simulink model "FlyingSheet_simulator"  (R2019b)
settings: Solver=VariableStepAuto  StartTime=0.0  StopTime=30  RelTol=1e-3
values from neighbouring files (symbols this model uses):
  p =     [ds.mat]    (also in vxs.mat)
undefined symbols (not defined in the file or in its folder): quatnormalize
libraries: aerolibutil x24, simulink x14, sharedtransform x6, vrlib x4, sharedutil x3, simulink_extras x2, dspsrcs4 x1, aerolibanim x1, aerolibanimutils x1
(part 1 of 2)
settings Model: NumberOfSteps=10000  Creator=Robert  LastModifiedBy=Robert
settings DataIOCC: ReturnWorkspaceOutputs=off
settings DebuggingCC: ArithmeticOperatorsInVariantConditions=warning
settings SFSimCC: CustomCodeUndefinedFunction=UseInterfaceOnly

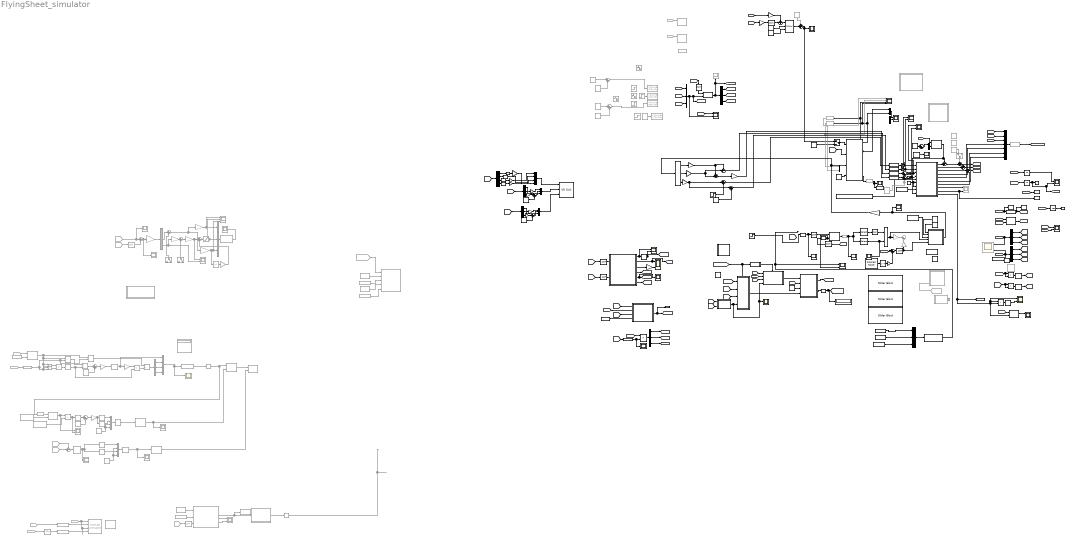
== system FlyingSheet_simulator ==
  note: Awesome Animation
  note: Green - FlyMode
      | Red = HoverMode
  note: ANimations above do not work bc gimbal lock.
  note: Thrust PID (Currently manages altitude velocity)
  note: Waypoint system,
      | Line generation,
      | reference velocity generation
  note: 0.01
  note: References are now generated in the
      |  block below this one. If you want to
      | choose your own referrence velocities
      | connect the "to" blocks with reference
      | signals here instead.
  note: Initial orientation; third argument multiplied
      | by 0 means bf and wf are aligned at start,
      | multiplied by 1 means tilted up 90 deg to
      | hiver mode at start,
  note: Man I really like playin with different reference
      | velocities, it is fun inducing crashes of the drone
  note: This is an ad-hoc way of generating a reference quaternion that can reject disturbances.
      | If body frame z-velocity is off, adjust pitch. If body frame y-velocity is off adjust yaw and roll. (This should be changed somehow)
      | body frame x-velocity is taken by another PID for joint thrust up to the right.
  note: THE HOLY GRAIL
  note: Reference velocities, set in wf
  note: For plotting trajectory in matlab
  note: Emil Fresk paper on quaternion control
  note: Rotate vector from bf to wf given q_wf
  note: Switch q between bf and wf
  note: Rotate vector from wf to bf given q_bf
  note: Matlab equivalent:
      |
      | v_wf = quatrotate(q_wf, v_bf)
      |
      |
      |
      |
      | v_bf = quatrotate(q_bf, v_wf)
      |
      |
      |
      |
      |
      |
      |
      | q_conj = quatconj(q)
  note: Adjust pitch to keep vzr_wf
  note: make sure wings horisontal
  note: See that q_uv block above? This block arangement does the same, but without calling a custom matlab block which may slow down sims.
  note: Try to figure out how to set our reference quaternion as a function of reference velocity vector, current velocity, etc.
  Abs : Abs  Commented=on
  Acos : Trigonometry  Commented=on  Operator=acos
  Acos1 : Trigonometry  Operator=acos
  AdHoc2 : MATLAB Function  Commented=on  TreatAsAtomicUnit=on
  Asin : Trigonometry  Operator=asin
  Asin1 : Trigonometry  Operator=asin
  Asin2 : Trigonometry  Operator=asin
  Band-Limited White Noise : simulink/Sources/Band-Limited White Noise  Commented=on  Cov=[0.01]  Ts=0.2  seed=[23343]
  Band-Limited White Noise1 : simulink/Sources/Band-Limited White Noise  Commented=on  Cov=[0.01]  Ts=0.1  seed=[23342]
  Band-Limited White Noise2 : simulink/Sources/Band-Limited White Noise  Commented=on  Cov=[0.01]  Ts=0.1  seed=[23341]
  Band-Limited White Noise3 : simulink/Sources/Band-Limited White Noise  Cov=[0.03]  Ts=1  seed=[23341]
  Colored Noise : dspsrcs4/Colored Noise  Color=pink  InverseFrequencyPower=1  BoundedOutput=on  NumChannels=3  OutputDataType=single  SamplesPerFrame=1  SampleTime=1/120  RandomStream=mt19937ar with seed  Seed=67  SimulateUsing=Interpreted execution
      settings: SourceProductName=DSP System Toolbox  SourceProductBaseCode=DS
  Constant : Constant  Commented=on  Value=-0.195
  Constant1 : Constant  Commented=on  Value=-5
  Constant10 : Constant  Value=6
  Constant11 : Constant  Value=15
  Constant12 : Constant  Value=0
  Constant13 : Constant  Value=18  SampleTime=p.Ts
  Constant14 : Constant  Commented=on  Value=pi/2
  Constant15 : Constant  Commented=on  Value=0
  Constant16 : Constant  Commented=on  Value=0
  Constant17 : Constant  Value=[4,8,2]'
  Constant18 : Constant  Value=0
  Constant{19..20,25..26} (4 alike) : Constant  Commented=on  Value=0.005  SampleTime=p.Ts
  Constant2 : Constant  Value=quatnormalize([cosd(60/2),0, 1*sind(60/2),0])  VectorParams1D=off
  Constant21 : Constant  Value=0
  Constant22 : Constant  Value=10
  Constant23 : Constant  Commented=on  Value=0.005*6  SampleTime=p.Ts
  Constant24 : Constant  Commented=on  Value=0.005*3  SampleTime=p.Ts
  Constant27 : Constant  Value=10
  Constant28 : Constant  Value=[4,4,10]  VectorParams1D=off
  Constant29 : Constant
  Constant3 : Constant  Value=290
  Constant30 : Constant  Value=600  SampleTime=p.Ts
  Constant31 : Constant  Value=0.6
  Constant32 : Constant  Value=0.1
  Constant4 : Constant  Commented=on  Value=-6
  Constant5 : Constant  Value=0.11  SampleTime=p.Ts
  Constant6 : Constant  Commented=on  Value=5 + 0*500
  Constant7 : Constant  Commented=on
  Constant8 : Constant
  Constant9 : Constant  Commented=on  Value=0
  Cos : Trigonometry  Commented=on  Operator=cos
  Cos1 : Trigonometry  Commented=on  Operator=cos
  Cross Product1 : vrlib/Utilities/Cross Product  Commented=on
      settings: SourceProductBaseCode=VR
  Dashboard : Subsystem
  Delay : Delay  DelayLength=1
  Demux{,2..4,6..7,10} (7 alike) : Demux  Outputs=3
  Demux1 : Demux  Commented=on  Outputs=3
  Demux5 : Demux  Commented=on  Outputs=3
  Demux8 : Demux
  Display : Display  Commented=on
  Display1 : Display
  Divide : Product  Commented=on  Inputs=*/
  Divide1 : Product  Commented=on  Inputs=*/
  Dot Product{1..3,6} (4 alike) : DotProduct  Commented=on  InputSameDT=on  OutDataTypeStr=Inherit: Inherit via internal rule
  Dot Product4 : DotProduct  InputSameDT=on  OutDataTypeStr=Inherit: Inherit via internal rule
  Dot Product5 : DotProduct  InputSameDT=on  OutDataTypeStr=Inherit: Inherit via internal rule
  Dot Product7 : DotProduct  InputSameDT=on  OutDataTypeStr=Inherit: Inherit via internal rule
  FlyVecAdjust : MATLAB Function  TreatAsAtomicUnit=on
  From : From  Commented=on  GotoTag=vr_bf
  From26 : From  Commented=on  GotoTag=q_wf
  From27 : From  Commented=on  GotoTag=vr_wf
  From28 : From  Commented=on  GotoTag=v_bf
  From33 : From  Commented=on  GotoTag=vz_wf
  From34 : From  Commented=on  GotoTag=vzr_wf
  From36 : From  Commented=on  GotoTag=r_wf
  From40 : From  Commented=on  GotoTag=q_ref
  From41 : From  Commented=on  GotoTag=r_wf
  From42 : From  Commented=on  GotoTag=q_bf
  From45 : From  Commented=on  GotoTag=hovermode
  From46 : From  Commented=on  GotoTag=hovermode
  From60 : From  Commented=on  GotoTag=q_bf
  From61 : From  Commented=on  GotoTag=q_wf
  Gain : Gain  Commented=on  Gain=30
  Gain1 : Gain  Commented=on  Gain=7.5
  Gain10 : Gain  Gain=750
  Gain11 : Gain  Commented=on  Gain=0.1
  Gain12 : Gain  Commented=on  Gain=0.02
  Gain13 : Gain
  Gain{14,16,19..20,23..27} (9 alike) : Gain  Gain=-1
  Gain15 : Gain  Commented=on  Gain=0.5
  Gain17 : Gain  Gain=10
  Gain2 : Gain  Commented=on  Gain=5
  Gain22 : Gain  Gain=-2
  Gain28 : Gain  Gain=0.1
  Gain3 : Gain
  Gain4 : Gain  Gain=0.01
  Gain5 : Gain  Commented=on  Gain=-1
  Gain6 : Gain  Commented=on  Gain=0
  Gain7 : Gain  Commented=on  Gain=0.5
  Gain8 : Gain  Commented=on  Gain=0.5
  Gain9 : Gain  Commented=on  Gain=2
  Integrator : Integrator
  Integrator1 : Integrator
  Integrator2 : Integrator
  Inveter : Subsystem
  MATLAB Animation : aerolibanim/MATLAB Animation  Tag=Matlab Animation 6 DOF  Commented=on  Vehicles=2  Geometries={'astredwedge.mat',a}  BoundingBoxCoordinates=[-50,50,-50,50,-50,50]  CameraOffset=[-150,0,0]  CameraViewAngle=3  SampleTime=0.05  FigurePosition=[962,42,958,461]
      settings: SourceProductName=Aerospace Blockset  SourceProductBaseCode=AE
  MATLAB Function : MATLAB Function  Commented=on  TreatAsAtomicUnit=on
  MATLAB Function1 : MATLAB Function  Commented=on  TreatAsAtomicUnit=on
  MATLAB Function11 : MATLAB Function  TreatAsAtomicUnit=on
  MATLAB Function12 : MATLAB Function  Commented=on  TreatAsAtomicUnit=on
  MATLAB Function2 : MATLAB Function  Commented=through  TreatAsAtomicUnit=on
  MATLAB Function3 : MATLAB Function  TreatAsAtomicUnit=on
  MATLAB Function5 : MATLAB Function  Commented=on  TreatAsAtomicUnit=on
  MATLAB Function7 : MATLAB Function  Commented=on  TreatAsAtomicUnit=on
  MATLAB Function9 : MATLAB Function  TreatAsAtomicUnit=on
  Manual Switch : ManualSwitch  Commented=on
  Manual Switch1 : ManualSwitch  Commented=on  CurrentSetting=0
  Manual Switch2 : ManualSwitch  Commented=on  CurrentSetting=0
  Manual Switch3 : ManualSwitch
  Multiply : Product
  Multiply1 : Product
  Multiply2 : Product  Commented=on
  Multiply3 : Product  Commented=on
  Mux : Mux  Inputs=7
  Mux1 : Mux  Commented=on  Inputs=3
  Mux{2,6,10,12,14} (5 alike) : Mux  Inputs=3
  Mux13 : Mux
  Mux3 : Mux  Inputs=2
  Mux4 : Mux  Inputs=2
  Mux5 : Mux  Commented=on
  Mux7 : Mux  Inputs=2
  Mux8 : Mux  Commented=on
  Mux9 : Mux  Commented=on
  Normalize Vector : vrlib/Utilities/Normalize Vector  Commented=on  maxzero=0
      settings: SourceProductName=Simulink 3D Animation  SourceProductBaseCode=VR
  Normalize Vector1 : vrlib/Utilities/Normalize Vector  maxzero=0
      settings: SourceProductName=Simulink 3D Animation  SourceProductBaseCode=VR
  PID Controller : simulink/Continuous/PID Controller  Controller=PID  Form=Parallel  TimeDomain=Discrete-time  SampleTime=-1  IntegratorMethod=Forward Euler  FilterMethod=Forward Euler  ControllerParametersSource=internal  P=3  I=3  D=0  UseFilter=off  N=100  TunerSelectOption=Frequency Response Based  InitialConditionSource=external  InitialConditionForIntegrator=0  InitialConditionForFilter=0  DifferentiatorICPrevScaledInput=0  ExternalReset=none  TrackingMode=off  Kt=1  LimitOutput=on  UpperSaturationLimit=30  LowerSaturationLimit=0  LinearizeAsGain=on  AntiWindupMode=clamping  Kb=1  POutMin=[]  POutMax=[]  IOutMin=[]  IOutMax=[]  DOutMin=[]  DOutMax=[]  NOutMin=[]  NOutMax=[]  SumOutMin=[]  SumOutMax=[]  SaturationOutMin=[]  SaturationOutMax=[]  PParamMin=[]  PParamMax=[]  IParamMin=[]  IParamMax=[]  DParamMin=[]  DParamMax=[]  NParamMin=[]  NParamMax=[]  KbParamMin=[]  KbParamMax=[]  KtParamMin=[]  KtParamMax=[]  KbOutMin=[]  KbOutMax=[]  KtOutMin=[]  KtOutMax=[]  IntegratorOutMin=[]  IntegratorOutMax=[]  FilterOutMin=[]  FilterOutMax=[]  SumI1OutMin=[]  SumI1OutMax=[]  SumI2OutMin=[]  SumI2OutMax=[]  SumI3OutMin=[]  SumI3OutMax=[]  SumI4OutMin=[]  SumI4OutMax=[]  SumDOutMin=[]  SumDOutMax=[]  DifferentiatorOutMin=[]  DifferentiatorOutMax=[]  FilterDiffOutCoefMin=[]  FilterDiffOutCoefMax=[]  ReciprocalOutMin=[]  ReciprocalOutMax=[]  SumDenOutMin=[]  SumDenOutMax=[]  SumNumOutMin=[]  SumNumOutMax=[]  DivideOutMin=[]  DivideOutMax=[]  IntegratorContinuousStateAttributes=''  IntegratorStateMustResolveToSignalObject=off  IntegratorRTWStateStorageClass=Auto  FilterContinuousStateAttributes=''  FilterStateMustResolveToSignalObject=off  FilterRTWStateStorageClass=Auto  ParallelPVariant=InternalParameters  IdealPVariant=Disabled  IVariant=InternalParameters  DVariant=InternalParameters  IntegratorVariant=Discrete  SatVariant=Enabled  AWVariant=DiscClampingParallel  PCopyVariant=Disabled  TRVariant=Disabled  FdbkBlocksVariant=Forward  IdealPFdbkVariant=Disabled  SatFdbkVariant=Disabled  DerivativeFilterVariant=Differentiator  NVariant=Passthrough  NCopyVariant=Disabled_SignalSpec  FilterICVariant=ExternalICs  IntegratorICVariant=ExternalICs  ExternalResetVariant=Disabled  TRSumVariant=Passthrough  SumFdbkVariant=Disabled  SumVariant=Sum_PID
  PID Controller5 : simulink/Continuous/PID Controller  Commented=on  Controller=PID  Form=Parallel  TimeDomain=Continuous-time  SampleTime=-1  IntegratorMethod=Forward Euler  FilterMethod=Forward Euler  ControllerParametersSource=internal  P=0.04*2  I=0  D=0  UseFilter=on  N=100  TunerSelectOption=Transfer Function Based (PID Tuner App)  InitialConditionSource=internal  InitialConditionForIntegrator=0  InitialConditionForFilter=0  DifferentiatorICPrevScaledInput=0  ExternalReset=none  TrackingMode=off  Kt=1  LimitOutput=off  UpperSaturationLimit=inf  LowerSaturationLimit=-inf  LinearizeAsGain=on  AntiWindupMode=none  Kb=1  POutMin=[]  POutMax=[]  IOutMin=[]  IOutMax=[]  DOutMin=[]  DOutMax=[]  NOutMin=[]  NOutMax=[]  SumOutMin=[]  SumOutMax=[]  SaturationOutMin=[]  SaturationOutMax=[]  PParamMin=[]  PParamMax=[]  IParamMin=[]  IParamMax=[]  DParamMin=[]  DParamMax=[]  NParamMin=[]  NParamMax=[]  KbParamMin=[]  KbParamMax=[]  KtParamMin=[]  KtParamMax=[]  KbOutMin=[]  KbOutMax=[]  KtOutMin=[]  KtOutMax=[]  IntegratorOutMin=[]  IntegratorOutMax=[]  FilterOutMin=[]  FilterOutMax=[]  SumI1OutMin=[]  SumI1OutMax=[]  SumI2OutMin=[]  SumI2OutMax=[]  SumI3OutMin=[]  SumI3OutMax=[]  SumI4OutMin=[]  SumI4OutMax=[]  SumDOutMin=[]  SumDOutMax=[]  DifferentiatorOutMin=[]  DifferentiatorOutMax=[]  FilterDiffOutCoefMin=[]  FilterDiffOutCoefMax=[]  ReciprocalOutMin=[]  ReciprocalOutMax=[]  SumDenOutMin=[]  SumDenOutMax=[]  SumNumOutMin=[]  SumNumOutMax=[]  DivideOutMin=[]  DivideOutMax=[]  IntegratorContinuousStateAttributes=''  IntegratorStateMustResolveToSignalObject=off  IntegratorRTWStateStorageClass=Auto  FilterContinuousStateAttributes=''  FilterStateMustResolveToSignalObject=off  FilterRTWStateStorageClass=Auto  ParallelPVariant=InternalParameters  IdealPVariant=Disabled  IVariant=InternalParameters  DVariant=InternalParameters  IntegratorVariant=Continuous  SatVariant=Disabled  AWVariant=Passthrough  PCopyVariant=Disabled  TRVariant=Disabled  FdbkBlocksVariant=Forward  IdealPFdbkVariant=Disabled  SatFdbkVariant=Disabled  DerivativeFilterVariant=ContFilter  NVariant=InternalParameters  NCopyVariant=Disabled  FilterICVariant=InternalICsFilter  IntegratorICVariant=InternalICs  ExternalResetVariant=Disabled  TRSumVariant=Passthrough  SumFdbkVariant=Disabled  SumVariant=Sum_PID
  Pulse Generator : DiscretePulseGenerator  Commented=on  PulseType=Time based  Amplitude=12  Period=50  PulseWidth=50
  Pulse Generator1 : DiscretePulseGenerator  Commented=on  PulseType=Time based  Amplitude=8  Period=60  PulseWidth=50  PhaseDelay=30
  Quaternion Conjugate{1..2,4..6,9} (6 alike) : aerolibutil/Quaternion Conjugate  Commented=on
      settings: SourceProductName=Aerospace Blockset  SourceProductBaseCode=AE
  Quaternion Conjugate10 : aerolibutil/Quaternion Conjugate  Commented=through
      settings: SourceProductName=Aerospace Blockset  SourceProductBaseCode=AE
  Quaternion Conjugate3 : aerolibutil/Quaternion Conjugate
      settings: SourceProductName=Aerospace Blockset  SourceProductBaseCode=AE
  Quaternion Conjugate7 : aerolibutil/Quaternion Conjugate
      settings: SourceProductName=Aerospace Blockset  SourceProductBaseCode=AE
  Quaternion Conjugate8 : aerolibutil/Quaternion Conjugate
      settings: SourceProductName=Aerospace Blockset  SourceProductBaseCode=AE
  Quaternion Multiplication : aerolibutil/Quaternion Multiplication
  Quaternion Multiplication1 : aerolibutil/Quaternion Multiplication  Commented=on
  Quaternion Multiplication2 : aerolibutil/Quaternion Multiplication  Commented=on
  Quaternion Normalize : sharedutil/Quaternion Normalize  Commented=on  aMode=aMode
      settings: SourceProductName=Aerospace Blockset  SourceProductBaseCode=AE
  Quaternion Normalize1 : sharedutil/Quaternion Normalize  Commented=on  aMode=aMode
      settings: SourceProductName=Aerospace Blockset  SourceProductBaseCode=AE
  Quaternion Normalize2 : sharedutil/Quaternion Normalize  Commented=on  aMode=aMode
      settings: SourceProductName=Aerospace Blockset  SourceProductBaseCode=AE
  Quaternion Rotation{1,4,6,8} (4 alike) : aerolibutil/Quaternion Rotation
  Quaternion Rotation{2..3,5,7} (4 alike) : aerolibutil/Quaternion Rotation  Commented=on
  Quaternions to Rotation Angles1 : sharedtransform/Quaternions to Rotation Angles  Commented=on  rotationOrder=XYZ  aMode=aMode
      settings: SourceProductBaseCode=AE
  Quaternions to Rotation Angles2 : sharedtransform/Quaternions to Rotation Angles  Commented=on  rotationOrder=XYZ  aMode=aMode
      settings: SourceProductBaseCode=AE
  Rate Limiter : RateLimiter  SampleTimeMode=inherited  InitialCondition=0.01
  Rotation Angles to Quaternions : sharedtransform/Rotation Angles to Quaternions  Commented=on  rotationOrder=ZYX  aMode=aMode
      settings: SourceProductName=Aerospace Blockset  SourceProductBaseCode=AE
  Rotation Angles to Quaternions1 : sharedtransform/Rotation Angles to Quaternions  rotationOrder=ZYX  aMode=aMode
      settings: SourceProductName=Aerospace Blockset  SourceProductBaseCode=AE
  Saturation : Saturate  UpperLimit=1000  LowerLimit=0
  Saturation1 : Saturate  UpperLimit=1000  LowerLimit=0
  Saturation2 : Saturate
  Saturation3 : Saturate
  Saturation4 : Saturate  Commented=through
  Saturation6 : Saturate  Commented=on  UpperLimit=1  LowerLimit=-1
  Scope{,2,6,10,19,23} (6 alike) : Scope  NumInputPorts=2
  Scope{1,11..12,15,18} (5 alike) : Scope  Commented=on  NumInputPorts=2
  Scope{4..5,13,20,24..26,28,34..35} (10 alike) : Scope
  Scope{3,8..9,14,17,21} (6 alike) : Scope  Commented=on
  Scope16 : Scope  Commented=on  NumInputPorts=3
  Scope27 : Scope  NumInputPorts=4
  Selector : Selector  IndexMode=Zero-based  InputPortWidth=4  IndexOptions=Index vector (dialog)  Indices=[0 ]  OutputSizes=1
  Selector1 : Selector  IndexMode=Zero-based  InputPortWidth=4  IndexOptions=Index vector (dialog)  Indices=[1:3]  OutputSizes=1
  Sign : Signum
  Signal Specification{,1..3} (4 alike) : SignalSpecification  Dimensions=1
  Signal Specification4 : SignalSpecification  Commented=through  Dimensions=14
  Signal Specification5 : SignalSpecification  Commented=through  Dimensions=[1 3]
  Simulation Pace : aerolibanimutils/Simulation Pace  Commented=on  SimulationPace=1  SleepMode=Auto  OutputPaceError=off  SampleTime=1/30
  Sin : Trigonometry  Commented=on
  Sin1 : Trigonometry  Commented=on
  Sine Wave : Sin  Commented=on  Amplitude=-2  Frequency=1/15  Phase=pi/2  SampleTime=0
  Sine Wave1 : Sin  Commented=on  Amplitude=-8  Frequency=1/20  SampleTime=0
  Sine Wave2 : Sin  Commented=on  Amplitude=10  Frequency=1/45  SampleTime=0
  Slider : SliderBlock  ScaleMin=-3.1400000000000001  ScaleMax=3.1400000000000001
  Slider1 : SliderBlock  ScaleMin=-3.1400000000000001  ScaleMax=3.1400000000000001
  Slider2 : SliderBlock  ScaleMin=-3  ScaleMax=3
  Sqrt : Sqrt  Commented=on  SaturateOnIntegerOverflow=on
  Sqrt1 : Sqrt  Commented=on  SaturateOnIntegerOverflow=on
  Sqrt2 : Sqrt  SaturateOnIntegerOverflow=on
  Sqrt3 : Sqrt  SaturateOnIntegerOverflow=on
  Sqrt4 : Sqrt  SaturateOnIntegerOverflow=on
  State-Space1 : StateSpace  Commented=on  A=-1/5  B=1/5  D=0  InitialCondition=0
  State-Space2 : StateSpace  Commented=on  A=-1/15  B=1/15  D=0  InitialCondition=0
  State-Space3 : StateSpace  Commented=on  A=-1/15  B=1/15  D=0  InitialCondition=0
  State-Space4 : StateSpace  Commented=on  A=-1/15  B=1/15  D=0  InitialCondition=0
  Step : Step  Time=20  Before=[cos(pi/4),0,sin(pi/4),0]  After=[1,0,0,0]  SampleTime=0
  Step1 : Step  Commented=on  Time=20  After=-10  SampleTime=0
  Step2 : Step  Commented=on  Time=100  After=5  SampleTime=0
  Step3 : Step  Commented=on  Time=30  Before=-1  After=0  SampleTime=0
  Step4 : Step  Commented=on  Time=60  After=18  SampleTime=0
  Step5 : Step  Time=5  Before=600  After=580  SampleTime=0
  Sum : Sum  Commented=on  Inputs=|--
  Sum{1..2,6,17..18,23,25} (7 alike) : Sum  Inputs=|++
  Sum10 : Sum  Commented=on  Inputs=|+-
  Sum{5,11..13,20} (5 alike) : Sum  Inputs=++|
  Sum{3,7..9,14..15} (6 alike) : Sum  Commented=on  Inputs=|++
  Sum16 : Sum  Inputs=-+|
  Sum19 : Sum  Inputs=-+|
  Sum21 : Sum  Commented=on  Inputs=|+-
  Sum22 : Sum  Commented=on  Inputs=-+|
  Sum24 : Sum  Inputs=|-+
  Sum4 : Sum  Inputs=+-|
  TailSitter : Subsystem
  To Workspace : ToWorkspace  VariableName=r  SaveFormat=Timeseries  SampleTime=p.Ts_log
  To Workspace1 : ToWorkspace  VariableName=q_bf  SaveFormat=Timeseries  SampleTime=p.Ts_log
  To Workspace10 : ToWorkspace  VariableName=eq_gains  SaveFormat=Timeseries  SampleTime=-1
  To Workspace2 : ToWorkspace  VariableName=v_bf  SaveFormat=Timeseries  SampleTime=p.Ts_log
  To Workspace3 : ToWorkspace  VariableName=a_bf  SaveFormat=Timeseries  SampleTime=p.Ts_log
  To Workspace4 : ToWorkspace  VariableName=q_wf  SaveFormat=Timeseries  SampleTime=p.Ts_log
  To Workspace5 : ToWorkspace  VariableName=rr  SaveFormat=Timeseries  SampleTime=p.Ts_log
  To Workspace6 : ToWorkspace  VariableName=gravity_bf  SaveFormat=Timeseries  SampleTime=p.Ts_log
  To Workspace7 : ToWorkspace  VariableName=v_wf  SaveFormat=Timeseries  SampleTime=p.Ts_log
  To Workspace8 : ToWorkspace  VariableName=refvec  SaveFormat=Timeseries  SampleTime=p.Ts_log
  To Workspace9 : ToWorkspace  Commented=on  VariableName=refvec1  SaveFormat=Timeseries  SampleTime=p.Ts_log
  TorqueTranslator : MATLAB Function  TreatAsAtomicUnit=on
  Torque_FL : MATLAB Function  Commented=on  TreatAsAtomicUnit=on
  Transfer Fcn First Order : simulink/Discrete/Transfer Fcn First Order  Commented=on  PoleZ=0.95  ICPrevOutput=0.0  DoSatur=off
      settings: SourceProductName=Simulink
  Transfer Fcn First Order1 : simulink/Discrete/Transfer Fcn First Order  Commented=on  PoleZ=0.95  ICPrevOutput=0.0  DoSatur=off
      settings: SourceProductName=Simulink
  Transpose : Math  Operator=transpose  SignedPower=off  SaturateOnIntegerOverflow=on
  VR Sink : vrlib/VR Sink  InstantiateOnLoad=on  SampleTime=0.05  ViewEnable=on  RemoteChange=off  RemoteView=off  FieldsWritten=Plane.rotation.4.1.1.double#Plane.translation.3.1.1.double#Block.translation.3.1.1.double  WorldFileName=vrtkoff_hud.wrl  WorldDescription=VR Plane Take-Off with HUD Text  AutoView=on  VideoDimensions=[600 860]  AllowVariableSize=off  FigureProperties="{'Position', 'Name', 'Viewpoint', 'CameraBound', 'CameraDirection', 'CameraPosition', 'CameraUpVector', 'ZoomFactor', 'Antialiasing', 'Headlight', 'Lighting', 'NavPanel', 'Sound', 'StatusBar', 'Stereo3D', 'Stereo3DCameraOffset', 'Stereo3DHIT', 'ToolBar', 'Textures', 'Transparency', 'Triad', 'Wireframe', 'NavZones', 'NavMode', 'NavSpeed', 'CaptureFileFormat', 'CaptureFileName', 'Record2DCompressMethod', 'Record2DCompressQuality', 'Record2D', 'Record2DFileName', 'Record2DFPS'; [9.6200000000000000e+02   8.4000000000000000e+01   9.5800000000000000e+02   3.8400000000000000e+02], 'VR Plane Take-Off with HUD Text', 'Observe Plane', 'on', [-4.2787674820401950e-01  -1.1740140648252211e-01   8.9617989159671219e-01], [1.7670687419247848e+01   7.2326607669184346e+00  -4.4972995858895132e+01], [4.6581268753260749e-03   9.9122851822676961e-01   1.3207697190645110e-01], [1.0000000000000000e+00], 'off', 'on', 'on', 'halfbar', 'on', 'on', 'off', [1.0000000149011612e-01], [0.0000000000000000e+00], 'on', 'on', 'on', 'none', 'off', 'off', 'fly', 'normal', 'tif', '%f_anim_%n.tif', 'auto', [7.5000000000000000e+01], 'off', '%f_anim_%n.avi', 'auto'}"
      settings: SourceProductBaseCode=VR
  Zero-Order Hold{,1,4..5,7..9} (7 alike) : ZeroOrderHold  SampleTime=p.Ts
  Zero-Order Hold10 : ZeroOrderHold  Commented=on  SampleTime=p.Ts
  Zero-Order Hold2 : ZeroOrderHold  Commented=on  SampleTime=p.Ts
  Zero-Order Hold6 : ZeroOrderHold  Commented=on  SampleTime=p.Ts
  bodyfrme : Scope  NumInputPorts=2
  gravity : Scope  NumInputPorts=2
  gravity_wf_convertedfrombf : Scope  NumInputPorts=2
  linegenerator : MATLAB Function  TreatAsAtomicUnit=on
  linegenerator1 : MATLAB Function  Commented=on  TreatAsAtomicUnit=on
  pitch : Constant  Value=0
  q_fly_generator : Subsystem
  q_hover_generator : Subsystem
  roll : Constant  Value=0
  u_deltas : Scope  NumInputPorts=2
  u_omegas : Scope  NumInputPorts=2
  v_isnit : Constant  Value=[0, 0,0]
  "v_ref_bf_attctrl " : Scope  Commented=on
  vr-v : Scope  Commented=on
  x_bf : Constant  Commented=on  Value=[1,0,0]
  y_bf : Constant  Commented=on  Value=[0,1,0]
  yaw : Constant  Value=0
  z_wf : Constant  Commented=on  Value=[0,0,1]
  wires:
  Selector1/1 -> Multiply/2, Scope4/1  "axiserr"
  Selector/1 -> Sign/1  "q0"
  Sign/1 -> Multiply/1  "rotdir"
  Gain1/1 -> Sum/2
  Sum5/1 -> Manual Switch3/1, Scope13/1  "u_EnginePower"
  Constant3/1 -> TailSitter/7(omegaR_init), TailSitter/6(omegaL_init)
  Sum11/1 -> [v_bf]  "v"
  TailSitter/8(wdot) -> Scope1/1  "wdot"
  TailSitter/9(vdot) -> To Workspace3/1, Scope1/2  "vdot"
  Integrator/1 -> [r_wf], Scope2/2, To Workspace/1  "r_wf"
  [v_wf] -> Integrator/1
  v_isnit/1 -> TailSitter/8(v_init)
  Sum4/1 -> PID Controller/1
  PID Controller/1 -> Sum5/2
  Constant6/1 -> Sum5/1
  Multiply/1 -> Gain/1, MATLAB Function11/4(angErr)
  [vzr_wf] -> Gain19/1  "vxr_bf"
  Saturation/1 -> TailSitter/2(u_omegaR), u_omegas/2
  Saturation1/1 -> u_omegas/1, TailSitter/1(u_omegaL)
  TailSitter/3(q) -> Sum13/2
  Mux2/1 -> Scope10/2, [vr_wf], Quaternion Rotation1/2  "vref"
  Quaternion Rotation1/1 -> Demux2/1, [vr_bf], Scope9/1
  Demux2/3 -> [vzr_bf]
  Demux2/2 -> [vyr_bf]
  Demux2/1 -> [vxr_bf]
  Zero-Order Hold7/1 -> Sum4/2  "vx_bf"
  [v_wf] -> Scope10/1  "v_wf"
  [q_bf] -> Zero-Order Hold4/1
  [q_bf] -> To Workspace1/1, Quaternion Conjugate3/1
  Quaternion Conjugate3/1 -> To Workspace4/1, [q_wf]
  [vxr_wf] -> Mux2/1
  [vyr_wf] -> Mux2/2
  [vzr_wf] -> Mux2/3
  [q_wf] -> Quaternion Rotation4/1
  Quaternion Rotation4/1 -> [v_wf]
  [v_bf] -> Quaternion Rotation4/2
  TailSitter/2(w) -> Sum12/2  "w"
  Demux/1 -> [vx_bf]
  Demux/3 -> [vz_bf]
  Demux/2 -> [vy_bf]
  [v_bf] -> Scope11/1, Demux/1
  Demux4/2 -> [vy_wf]
  Demux4/3 -> [vz_wf]
  Demux4/1 -> [vx_wf]
  [v_wf] -> To Workspace7/1, Scope11/2, Demux4/1
  [v_bf] -> To Workspace2/1
  [v_bf] -> Dot Product4/2, Dot Product4/1
  Sqrt2/1 -> [abs_v]
  [vr_wf] -> Integrator1/1
  Integrator1/1 -> Scope2/1  "r_ref_wf"
  [w_bf] -> Sum25/1
  [v_bf] -> bodyfrme/1  "v"
  [vr_bf] -> bodyfrme/2  "vr"
  [vr_wf] -> Integrator2/1
  Integrator2/1 -> To Workspace5/1  "r_wf"
  Dot Product4/1 -> Sqrt2/1
  Gain/1 -> Sum/1
  Constant2/1 -> TailSitter/5(initialOrientation)  "qerr_wf"
  [v_bf] -> Mux/1  "v"
  [w_bf] -> Mux/2  "w"
  [q_bf] -> Mux/3  "q"
  TailSitter/5(deltaL) -> Mux/4  "deltaL"
  TailSitter/4(deltaR) -> Mux/5  "deltaR"
  TailSitter/7(omegaL) -> Mux/6  "omegaL"
  TailSitter/6(omegaR) -> Mux/7  "omegaR"
  TorqueTranslator/1(u_omegaL) -> Mux3/2, Transfer Fcn First Order/1, Scope27/4  "uWL"
  TorqueTranslator/2(u_omegaR) -> Mux3/1, Scope27/3, Transfer Fcn First Order1/1
  Signal Specification/1 -> Saturation1/1
  Signal Specification1/1 -> Saturation/1
  Signal Specification2/1 -> Sum1/1
  Signal Specification3/1 -> Sum2/1
  Mux/1 -> Signal Specification4/1
  Sum1/1 -> Saturation2/1
  Signal Specification4/1 -> [states]
  Acos/1 -> Sum21/1
  y_bf/1 -> Dot Product6/2
  Multiply3/1 -> Divide1/2
  Sum22/1 -> PID Controller5/1
  Dot Product3/1 -> Divide/1
  Demux5/2 -> Mux5/3
  Quaternion Conjugate6/1 -> Scope3/1, Quaternion Normalize2/1
  Mux5/1 -> Scope17/1, Quaternion Normalize/1
  From33/1 -> Sum22/1
  Constant15/1 -> Mux8/3, Mux8/4
  Mux8/1 -> Quaternion Conjugate1/1
  Demux5/1 -> Mux5/2
  PID Controller5/1 -> Scope8/1, Cos1/1, Sin1/1
  From27/1 -> Normalize Vector/1  "v_wf"
  Cos1/1 -> Mux9/1
  Quaternion Rotation7/1 -> Scope12/1, Dot Product6/1  "zwf_bf"
  Constant16/1 -> Mux9/2, Mux9/4
  Quaternion Normalize1/1 -> Scope21/1, Quaternion Multiplication1/2
  Gain7/1 -> Sin/1, Cos/1
  Sum21/1 -> Gain7/1
  From34/1 -> Sum22/2
  Mux9/1 -> Quaternion Conjugate6/1
  Cos/1 -> Mux8/1
  Constant14/1 -> Sum21/2
  Sin/1 -> Mux8/2
  Quaternion Normalize2/1 -> Quaternion Multiplication2/2
  Multiply2/1 -> Sqrt/1
  Divide/1 -> Sum14/1
  Quaternion Conjugate1/1 -> Quaternion Normalize1/1
  Sin1/1 -> Mux9/3
  Sqrt1/1 -> Mux5/1, Gain9/1
  Quaternion Conjugate4/1 -> Quaternion Rotation7/1
  Normalize Vector/1 -> Cross Product1/2, Dot Product3/2, Dot Product2/1, Dot Product2/2  "v_wf"
  Quaternion Normalize/1 -> Quaternion Conjugate5/1  "qerr_wf"
  Gain8/1 -> Sqrt1/1
  Cross Product1/1 -> Divide1/1
  Divide1/1 -> Demux5/1
  From26/1 -> Quaternion Rotation5/1
  Sum14/1 -> Gain8/1
  z_wf/1 -> Quaternion Rotation7/2
  Dot Product6/1 -> Scope12/2, Acos/1  "cos(a)"
  Gain9/1 -> Multiply3/1
  Dot Product1/1 -> Multiply2/1
  Constant7/1 -> Sum14/2
  Dot Product2/1 -> Multiply2/2
  Sqrt/1 -> Multiply3/2, Divide/2
  Quaternion Rotation5/1 -> Dot Product3/1, Dot Product1/2, Dot Product1/1, Cross Product1/1  "bfx_wf"
  Demux5/3 -> Mux5/4
  x_bf/1 -> Quaternion Rotation5/2
  Quaternion Multiplication1/1 -> Quaternion Multiplication2/1
  Quaternion Conjugate5/1 -> Quaternion Conjugate4/1, Quaternion Multiplication1/1  "qerr_wf"
  Mux1/1 -> Rotation Angles to Quaternions/1
  From28/1 -> Zero-Order Hold2/1
  Sum10/1 -> vr-v/1, Gain11/1
  Demux1/3 -> Gain5/1, Scope15/2
  Gain5/1 -> Sum9/1
  Sum7/1 -> Gain12/1, Gain6/1
  Gain6/1 -> Scope16/1, Mux1/1
  Gain15/1 -> Sum15/1, Scope15/1
  Gain11/1 -> Demux1/1
  Saturation2/1 -> u_deltas/1, TailSitter/3(u_deltaL)
  Sum2/1 -> Saturation3/1
  Saturation3/1 -> u_deltas/2, TailSitter/4(u_deltaR)
  Constant/1 -> Sum1/2, Sum2/2  "udeltaL"
  Sum3/1 -> State-Space1/1
  Gain12/1 -> Abs/1, Scope16/3, Mux1/3
  Dot Product5/1 -> Sqrt3/1
  Sqrt3/1 -> [abs_vr]
  [vr_wf] -> Dot Product5/2, Dot Product5/1
  From/1 -> "v_ref_bf_attctrl "/1, Sum10/1
  Sum8/1 -> State-Space2/1
  Step4/1 -> State-Space4/1
  TailSitter/10(gravity) -> To Workspace6/1, gravity/1, Dot Product7/1, Quaternion Rotation8/2, Dot Product7/2  "g_bf"
  Dot Product7/1 -> Sqrt4/1
  [q_wf] -> Quaternion Rotation8/1
  Quaternion Rotation8/1 -> gravity_wf_convertedfrombf/1
  Pulse Generator1/1 -> Sum3/1
  Constant1/1 -> Sum3/2
  Pulse Generator/1 -> Sum8/1
  Constant4/1 -> Sum8/2
  Sqrt4/1 -> gravity/2  "abs g"
  [v_wf] -> Zero-Order Hold/1
  Demux3/1 -> [vxr_wf]
  Multiply1/1 -> Demux3/1
  Demux1/2 -> Sum7/1
  linegenerator/2(wpN) -> [wpN], Scope19/1
  ? -> Saturation4/1
  Sum9/1 -> Gain15/1
  [rspeed] -> Multiply1/1
  Saturation6/1 -> Scope16/2, Mux1/2
  Constant9/1 -> State-Space3/1
  TailSitter/1(v) -> Sum16/2  "v"
  Sum12/1 -> [w_bf]  "v"
  Sum13/1 -> [q_bf]  "v"
  Band-Limited White Noise/1 -> Manual Switch/1
  Manual Switch/1 -> Sum11/1
  Zero-Order Hold/1 -> linegenerator/1(v_wf)
  Zero-Order Hold1/1 -> linegenerator/2(r)
  Zero-Order Hold2/1 -> Sum10/2
  Zero-Order Hold4/1 -> Quaternion Rotation1/1
  Zero-Order Hold5/1 -> Gain1/1, MATLAB Function11/5(w)
  [vz_wf] -> Gain20/1  "vx_bf"
  Manual Switch1/1 -> Sum9/2
  Manual Switch2/1 -> Sum7/2
  Zero-Order Hold9/1 -> Quaternion Multiplication/1
  Rotation Angles to Quaternions/1 -> Scope14/1  "qerr_wf"
  Mux4/1 -> Scope/2
  Mux3/1 -> Scope/1
  Abs/1 -> Gain2/1
  Sum15/1 -> Saturation6/1
  Gain2/1 -> Sum15/2
  Quaternion Multiplication/1 -> Quaternion Conjugate10/1  "qerr_wf"
  Gain19/1 -> Sum4/1
  Gain20/1 -> Zero-Order Hold7/1
  Demux3/3 -> [vzr_wf]
  linegenerator/3(dist2wp) -> Gain4/1
  Demux3/2 -> [vyr_wf]
  [r_wf] -> Zero-Order Hold1/1
  linegenerator/5(vec2line) -> [vec2line], Scope34/1
  FlyVecAdjust/1(refvec) -> To Workspace8/1, [refvec]
  Normalize Vector1/1 -> Scope24/1, Multiply1/2
  Zero-Order Hold8/1 -> Quaternion Conjugate7/1
  Gain4/1 -> Scope19/2
  [q_wf] -> Zero-Order Hold8/1  "qerr_bf"
  Quaternion Conjugate7/1 -> Scope23/2, Quaternion Multiplication/2
  Quaternion Conjugate8/1 -> Scope25/1, Zero-Order Hold9/1  "qerr_bf"
  linegenerator1/4(wpN) -> Scope18/1
  Quaternion Conjugate9/1 -> ?  "qerr_bf"
  linegenerator1/3(refvec) -> To Workspace9/1, MATLAB Function7/1(refvec)
  linegenerator1/5(dist2wp) -> Scope18/2
  Constant19/1 -> linegenerator1/2(d2lcoeff)
  MATLAB Function7/1(qref) -> Quaternion Conjugate9/1
  Constant20/1 -> linegenerator1/1(max2l)
  From41/1 -> Zero-Order Hold10/1
  Zero-Order Hold10/1 -> linegenerator1/3(r)
  [vr_wf] -> MATLAB Function9/2(vr_wf)
  yaw/1 -> Mux6/1
  pitch/1 -> Mux6/2
  roll/1 -> Mux6/3
  Zero-Order Hold6/1 -> Quaternions to Rotation Angles2/1
  From42/1 -> Zero-Order Hold6/1  "qerr_bf"
  Quaternions to Rotation Angles1/1 -> MATLAB Animation/2
  Quaternions to Rotation Angles2/1 -> MATLAB Animation/4
  From40/1 -> Quaternions to Rotation Angles1/1
  From36/1 -> MATLAB Animation/3, MATLAB Animation/1
  [r_wf] -> Demux6/1
  Demux6/1 -> Mux12/3
  Demux6/2 -> Gain23/1
  Demux6/3 -> Gain14/1
  Sum6/1 -> Mux12/2
  [q_wf] -> Demux8/1
  Demux8/3 -> Asin1/1
  Demux8/4 -> Asin/1
  Demux8/1 -> Acos1/1
  Acos1/1 -> Gain22/1
  Gain23/1 -> Mux12/1
  Gain24/1 -> Mux13/1
  Gain25/1 -> Mux13/2
  Asin2/1 -> Mux13/3
  Gain22/1 -> Mux13/4
  Gain14/1 -> Sum6/1
  Constant22/1 -> Sum6/2
  Asin/1 -> Gain25/1
  Asin1/1 -> Gain24/1
  Demux8/2 -> Asin2/1
  Manual Switch3/1 -> TorqueTranslator/1(u_jointT)
  Constant13/1 -> Manual Switch3/2
  MATLAB Function9/1(q_ref) -> [q_ref]
  Delay/1 -> Display1/1, [hovermode]  "hovermode"
  From46/1 -> MATLAB Function5/3(hovermode)
  Constant24/1 -> MATLAB Function12/2(c_hov)
  Constant23/1 -> MATLAB Function12/3(max_hov)
  Constant26/1 -> MATLAB Function12/4(c_fly)
  Constant25/1 -> MATLAB Function12/5(max_fly)
  From45/1 -> MATLAB Function12/1(hovermode)
  Mux13/1 -> VR Sink/1
  Mux12/1 -> VR Sink/2
  linegenerator/6(wp_r) -> [wp_r]
  Gain26/1 -> Sum17/1
  Sum17/1 -> Mux14/2
  Demux10/1 -> Mux14/3
  [wp_r] -> Demux10/1
  Demux10/2 -> Gain27/1
  Demux10/3 -> Gain26/1
  Gain27/1 -> Mux14/1
  Constant27/1 -> Sum17/2
  Mux14/1 -> VR Sink/3
  Quaternion Conjugate10/1 -> Selector1/1, Selector/1, Scope35/1
  MATLAB Function11/1(taos) -> Scope5/1, Gain28/1
  linegenerator/4(linevec) -> [linevec]
  q_fly_generator/1(q_ref_fly) -> MATLAB Function9/1(q_fly)
  q_hover_generator/1(q_ref_hover) -> MATLAB Function9/4(q_hover)
  [hovermode] -> Inveter/1(bool), q_hover_generator/Enable
  [rspeed] -> FlyVecAdjust/1(rspeed)
  [vec2line] -> FlyVecAdjust/2(vec2line)
  [linevec] -> FlyVecAdjust/3(linevec)
  Constant5/1 -> FlyVecAdjust/4(d2lcoeff)
  [refvec] -> Normalize Vector1/1
  MATLAB Function9/2(hovermode) -> Delay/1  "hovermode"
  [vec2line] -> q_hover_generator/1(vec2line)
  [linevec] -> q_hover_generator/2(linevec)
  [q_bf] -> q_hover_generator/3(q_bf)
  [vr_wf] -> q_fly_generator/1(vr_wf)
  [vec2line] -> q_fly_generator/2(vec2line)
  [v_wf] -> q_fly_generator/3(v_wf)
  Inveter/1(~bool) -> q_fly_generator/Enable
  Constant10/1 -> MATLAB Function9/3(v_cutoff)
  MATLAB Function3/1(yaw) -> Scope20/1, q_fly_generator/4(current_heading), q_hover_generator/4(current_heading)
  Rate Limiter/1 -> Scope6/2, [rspeed]
  linegenerator/1(rspeed) -> Scope6/1, Rate Limiter/1
  [v_wf] -> MATLAB Function3/1(v_wf)
  [vr_wf] -> MATLAB Function3/2(vr_wf)
  Constant11/1 -> PID Controller/2
  Constant12/1 -> PID Controller/3
  Rotation Angles to Quaternions1/1 -> Scope23/1
  Mux6/1 -> Rotation Angles to Quaternions1/1
  Step/1 -> Quaternion Conjugate8/1
  Constant28/1 -> MATLAB Function11/3(axisgains)
  TorqueTranslator/5(equivalent_gains) -> Signal Specification5/1
  Signal Specification5/1 -> Scope26/1, To Workspace10/1
  [states] -> TorqueTranslator/2(states)
  Transfer Fcn First Order/1 -> Mux7/1, Scope27/2
  Transfer Fcn First Order1/1 -> Scope27/1, Mux7/2
  Constant18/1 -> TorqueTranslator/4(pitchoffset)
  Quaternion Rotation6/1 -> TailSitter/9(wind), Sum16/1
  Sum16/1 -> Sum11/2
  From60/1 -> Quaternion Rotation2/1
  From61/1 -> Quaternion Rotation3/1
  [q_bf] -> Quaternion Rotation6/1
  Constant21/1 -> Sum18/1
  Sum18/1 -> Mux10/1
  Band-Limited White Noise3/1 -> Scope28/1
  Mux10/1 -> Quaternion Rotation6/2
  Demux7/2 -> Gain16/1
  Demux7/1 -> Gain13/1
  Gain28/1 -> Demux7/1, TorqueTranslator/3(wdots)
  Sum23/1 -> Signal Specification/1
  Gain10/1 -> Sum24/1, Sum23/1
  Sum24/1 -> Signal Specification1/1
  Sum20/1 -> Gain3/1
  Sum19/1 -> Signal Specification2/1
  Gain3/1 -> Signal Specification3/1
  Constant30/1 -> Sum24/2
  Demux7/3 -> Gain10/1
  Gain13/1 -> Sum19/1, Sum20/1
  Gain16/1 -> Sum20/2, Sum19/2
  Constant31/1 -> MATLAB Function11/1(P)
  Constant32/1 -> MATLAB Function11/2(D)
  Step5/1 -> Sum23/2
  Colored Noise/1 -> Transpose/1
  Sum25/1 -> Zero-Order Hold5/1
  Gain17/1 -> Sum25/2
  Transpose/1 -> Gain17/1

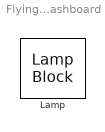
== system FlyingSheet_simulator/Dashboard ==
  Lamp : LampBlock

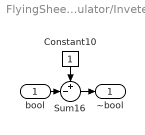
== system FlyingSheet_simulator/Inveter ==
  bool : Inport
  Constant10 : Constant
  Sum16 : Sum  Inputs=+-|
  ~bool : Outport  VectorParamsAs1DForOutWhenUnconnected=off
  wires:
  Constant10/1 -> Sum16/1
  bool/1 -> Sum16/2
  Sum16/1 -> ~bool/1

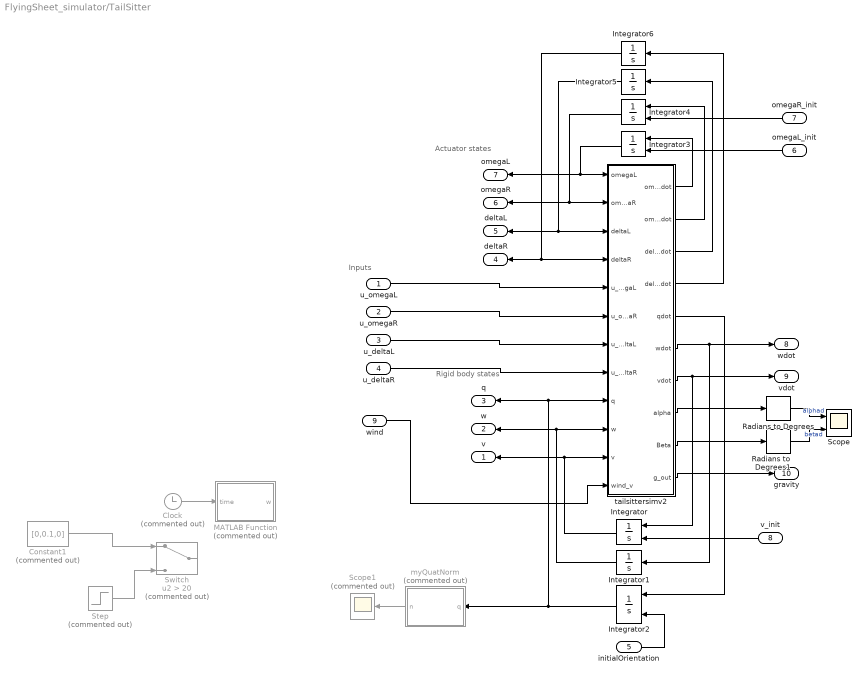
== system FlyingSheet_simulator/TailSitter ==
  note: Actuator
      | states
  note: Rigid
      | body
      | states
  note: Inputs
  u_omegaL : Inport
  u_omegaR : Inport  Port=2
  u_deltaL : Inport  Port=3
  u_deltaR : Inport  Port=4
  initialOrientation : Inport  Port=5
  omegaL_init : Inport  Port=6
  omegaR_init : Inport  Port=7
  v_init : Inport  Port=8
  wind : Inport  Port=9
  Clock : Clock  Commented=on
  Constant1 : Constant  Commented=on  Value=[0,0.1,0]
  Integrator : Integrator  InitialConditionSource=external  InitialCondition=[0,0,0]
  Integrator1 : Integrator  InitialCondition=[0,0,0]
  Integrator2 : Integrator  InitialConditionSource=external
  Integrator3 : Integrator  InitialConditionSource=external
  Integrator4 : Integrator  InitialConditionSource=external
  Integrator5 : Integrator
  Integrator6 : Integrator
  MATLAB Function : MATLAB Function  Commented=on  TreatAsAtomicUnit=on
  Radians to Degrees : simulink_extras/Transformations/Radians to Degrees
  Radians to Degrees1 : simulink_extras/Transformations/Radians to Degrees
  Scope : Scope  NumInputPorts=2
  Scope1 : Scope  Commented=on
  Step : Step  Commented=on  Time=10  Before=[0.1,0,0]  After=[0,0,0.1]  SampleTime=0
  Switch : Switch  Commented=on  Criteria=u2 > Threshold  Threshold=20
  myQuatNorm : MATLAB Function  Commented=on  TreatAsAtomicUnit=on
  tailsittersimv2 : MATLAB Function  TreatAsAtomicUnit=on
  v : Outport  VectorParamsAs1DForOutWhenUnconnected=off
  w : Outport  Port=2  VectorParamsAs1DForOutWhenUnconnected=off
  q : Outport  Port=3  VectorParamsAs1DForOutWhenUnconnected=off
  deltaR : Outport  Port=4  VectorParamsAs1DForOutWhenUnconnected=off
  deltaL : Outport  Port=5  VectorParamsAs1DForOutWhenUnconnected=off
  omegaR : Outport  Port=6  VectorParamsAs1DForOutWhenUnconnected=off
  omegaL : Outport  Port=7  VectorParamsAs1DForOutWhenUnconnected=off
  wdot : Outport  Port=8  PortDimensions=3  VectorParamsAs1DForOutWhenUnconnected=off
  vdot : Outport  Port=9  PortDimensions=3  VectorParamsAs1DForOutWhenUnconnected=off
  gravity : Outport  Port=10  PortDimensions=3  VectorParamsAs1DForOutWhenUnconnected=off
  wires:
  tailsittersimv2/7(vdot) -> Integrator/1, vdot/1
  tailsittersimv2/6(wdot) -> Integrator1/1, wdot/1
  tailsittersimv2/5(qdot) -> Integrator2/1
  Integrator2/1 -> tailsittersimv2/9(q), q/1, myQuatNorm/1(q)
  initialOrientation/1 -> Integrator2/2
  tailsittersimv2/1(omegaLdot) -> Integrator3/1
  Integrator3/1 -> tailsittersimv2/1(omegaL), omegaL/1
  tailsittersimv2/2(omegaRdot) -> Integrator4/1
  tailsittersimv2/3(deltaLdot) -> Integrator5/1
  tailsittersimv2/4(deltaRdot) -> Integrator6/1
  Integrator5/1 -> tailsittersimv2/3(deltaL), deltaL/1
  Integrator6/1 -> deltaR/1, tailsittersimv2/4(deltaR)
  Integrator4/1 -> tailsittersimv2/2(omegaR), omegaR/1
  omegaL_init/1 -> Integrator3/2
  omegaR_init/1 -> Integrator4/2
  u_omegaL/1 -> tailsittersimv2/5(u_omegaL)
  u_omegaR/1 -> tailsittersimv2/6(u_omegaR)
  u_deltaL/1 -> tailsittersimv2/7(u_deltaL)
  u_deltaR/1 -> tailsittersimv2/8(u_deltaR)
  tailsittersimv2/8(alpha) -> Radians to Degrees/1
  Radians to Degrees/1 -> Scope/1  "alphad"
  myQuatNorm/1(n) -> Scope1/1
  Integrator/1 -> tailsittersimv2/11(v), v/1
  Clock/1 -> MATLAB Function/1(time)
  Constant1/1 -> Switch/1
  Step/1 -> Switch/3
  Integrator1/1 -> tailsittersimv2/10(w), w/1
  v_init/1 -> Integrator/2
  tailsittersimv2/9(Beta) -> Radians to Degrees1/1
  Radians to Degrees1/1 -> Scope/2  "betad"
  tailsittersimv2/10(g_out) -> gravity/1
  wind/1 -> tailsittersimv2/12(wind_v)

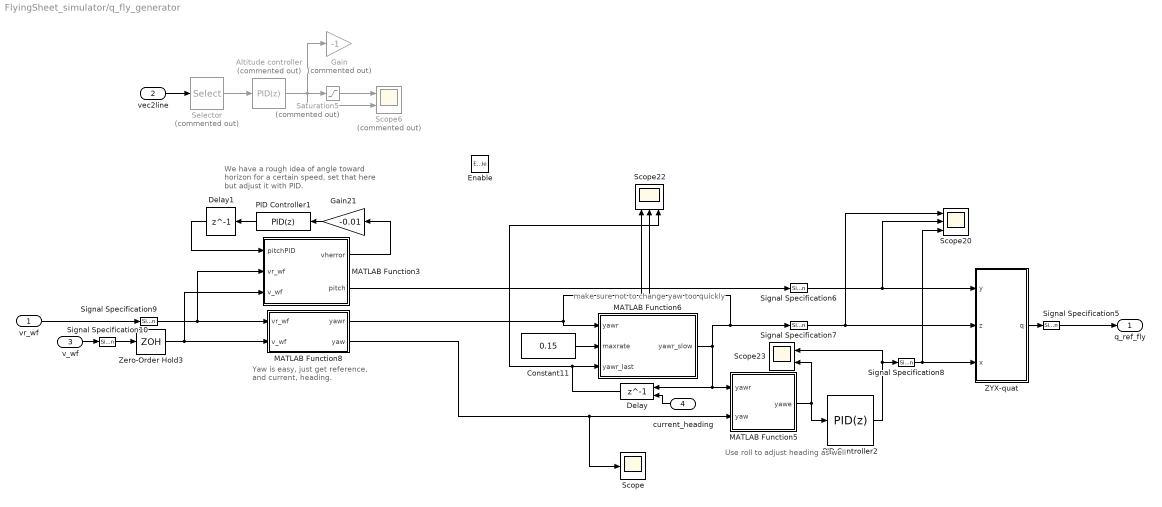
== system FlyingSheet_simulator/q_fly_generator ==
  note: Use roll to adjust heading as well
  note: make sure not to change yaw too quickly
  note: We have a rough idea of angle toward
      | horizon for a certain speed, set that here
      | but adjust it with PID.
  note: Yaw is easy, just get reference,
      | and current, heading.
  vr_wf : Inport
  vec2line : Inport  Port=2
  v_wf : Inport  Port=3
  current_heading : Inport  Port=4
  Enable : EnablePort  StatesWhenEnabling=reset
  Altitude controller : simulink/Continuous/PID Controller  Commented=on  Controller=PID  Form=Parallel  TimeDomain=Discrete-time  SampleTime=-1  IntegratorMethod=Forward Euler  FilterMethod=Forward Euler  ControllerParametersSource=internal  P=0.25  I=0  D=0.4*p.Ts  UseFilter=off  N=100  TunerSelectOption=Transfer Function Based (PID Tuner App)  InitialConditionSource=internal  InitialConditionForIntegrator=0  InitialConditionForFilter=0  DifferentiatorICPrevScaledInput=0  ExternalReset=none  TrackingMode=off  Kt=1  LimitOutput=off  UpperSaturationLimit=inf  LowerSaturationLimit=-inf  LinearizeAsGain=off  AntiWindupMode=none  Kb=1  POutMin=[]  POutMax=[]  IOutMin=[]  IOutMax=[]  DOutMin=[]  DOutMax=[]  NOutMin=[]  NOutMax=[]  SumOutMin=[]  SumOutMax=[]  SaturationOutMin=[]  SaturationOutMax=[]  PParamMin=[]  PParamMax=[]  IParamMin=[]  IParamMax=[]  DParamMin=[]  DParamMax=[]  NParamMin=[]  NParamMax=[]  KbParamMin=[]  KbParamMax=[]  KtParamMin=[]  KtParamMax=[]  KbOutMin=[]  KbOutMax=[]  KtOutMin=[]  KtOutMax=[]  IntegratorOutMin=[]  IntegratorOutMax=[]  FilterOutMin=[]  FilterOutMax=[]  SumI1OutMin=[]  SumI1OutMax=[]  SumI2OutMin=[]  SumI2OutMax=[]  SumI3OutMin=[]  SumI3OutMax=[]  SumI4OutMin=[]  SumI4OutMax=[]  SumDOutMin=[]  SumDOutMax=[]  DifferentiatorOutMin=[]  DifferentiatorOutMax=[]  FilterDiffOutCoefMin=[]  FilterDiffOutCoefMax=[]  ReciprocalOutMin=[]  ReciprocalOutMax=[]  SumDenOutMin=[]  SumDenOutMax=[]  SumNumOutMin=[]  SumNumOutMax=[]  DivideOutMin=[]  DivideOutMax=[]  IntegratorContinuousStateAttributes=''  IntegratorStateMustResolveToSignalObject=off  IntegratorRTWStateStorageClass=Auto  FilterContinuousStateAttributes=''  FilterStateMustResolveToSignalObject=off  FilterRTWStateStorageClass=Auto  ParallelPVariant=InternalParameters  IdealPVariant=Disabled  IVariant=InternalParameters  DVariant=InternalParameters  IntegratorVariant=Discrete  SatVariant=Disabled  AWVariant=Passthrough  PCopyVariant=Disabled  TRVariant=Disabled  FdbkBlocksVariant=Forward  IdealPFdbkVariant=Disabled  SatFdbkVariant=Disabled  DerivativeFilterVariant=Differentiator  NVariant=Passthrough  NCopyVariant=Disabled_SignalSpec  FilterICVariant=InternalICsDifferentiator  IntegratorICVariant=InternalICs  ExternalResetVariant=Disabled  TRSumVariant=Passthrough  SumFdbkVariant=Disabled  SumVariant=Sum_PID
  Constant11 : Constant  Value=0.15
  Delay : Delay  DelayLength=1  InitialConditionSource=Input port
      settings: InputPortMap=u0,p4
  Delay1 : Delay  DelayLength=1
  Gain : Gain  Commented=on  Gain=-1
  Gain21 : Gain  Gain=-0.01
  MATLAB Function3 : MATLAB Function  TreatAsAtomicUnit=on
  MATLAB Function5 : MATLAB Function  TreatAsAtomicUnit=on
  MATLAB Function6 : MATLAB Function  TreatAsAtomicUnit=on
  MATLAB Function8 : MATLAB Function  TreatAsAtomicUnit=on
  PID Controller1 : simulink/Continuous/PID Controller  Controller=PID  Form=Parallel  TimeDomain=Discrete-time  SampleTime=-1  IntegratorMethod=Forward Euler  FilterMethod=Forward Euler  ControllerParametersSource=internal  P=0  I=0.2  D=0  UseFilter=off  N=100  TunerSelectOption=Transfer Function Based (PID Tuner App)  InitialConditionSource=internal  InitialConditionForIntegrator=0  InitialConditionForFilter=0  DifferentiatorICPrevScaledInput=0  ExternalReset=none  TrackingMode=off  Kt=1  LimitOutput=on  UpperSaturationLimit=deg2rad(9)  LowerSaturationLimit=-deg2rad(9)  LinearizeAsGain=on  AntiWindupMode=clamping  Kb=1  POutMin=[]  POutMax=[]  IOutMin=[]  IOutMax=[]  DOutMin=[]  DOutMax=[]  NOutMin=[]  NOutMax=[]  SumOutMin=[]  SumOutMax=[]  SaturationOutMin=[]  SaturationOutMax=[]  PParamMin=[]  PParamMax=[]  IParamMin=[]  IParamMax=[]  DParamMin=[]  DParamMax=[]  NParamMin=[]  NParamMax=[]  KbParamMin=[]  KbParamMax=[]  KtParamMin=[]  KtParamMax=[]  KbOutMin=[]  KbOutMax=[]  KtOutMin=[]  KtOutMax=[]  IntegratorOutMin=[]  IntegratorOutMax=[]  FilterOutMin=[]  FilterOutMax=[]  SumI1OutMin=[]  SumI1OutMax=[]  SumI2OutMin=[]  SumI2OutMax=[]  SumI3OutMin=[]  SumI3OutMax=[]  SumI4OutMin=[]  SumI4OutMax=[]  SumDOutMin=[]  SumDOutMax=[]  DifferentiatorOutMin=[]  DifferentiatorOutMax=[]  FilterDiffOutCoefMin=[]  FilterDiffOutCoefMax=[]  ReciprocalOutMin=[]  ReciprocalOutMax=[]  SumDenOutMin=[]  SumDenOutMax=[]  SumNumOutMin=[]  SumNumOutMax=[]  DivideOutMin=[]  DivideOutMax=[]  IntegratorContinuousStateAttributes=''  IntegratorStateMustResolveToSignalObject=off  IntegratorRTWStateStorageClass=Auto  FilterContinuousStateAttributes=''  FilterStateMustResolveToSignalObject=off  FilterRTWStateStorageClass=Auto  ParallelPVariant=InternalParameters  IdealPVariant=Disabled  IVariant=InternalParameters  DVariant=InternalParameters  IntegratorVariant=Discrete  SatVariant=Enabled  AWVariant=DiscClampingParallel  PCopyVariant=Disabled  TRVariant=Disabled  FdbkBlocksVariant=Forward  IdealPFdbkVariant=Disabled  SatFdbkVariant=Disabled  DerivativeFilterVariant=Differentiator  NVariant=Passthrough  NCopyVariant=Disabled_SignalSpec  FilterICVariant=InternalICsDifferentiator  IntegratorICVariant=InternalICs  ExternalResetVariant=Disabled  TRSumVariant=Passthrough  SumFdbkVariant=Disabled  SumVariant=Sum_PID
  PID Controller2 : simulink/Continuous/PID Controller  Controller=PID  Form=Parallel  TimeDomain=Discrete-time  SampleTime=-1  IntegratorMethod=Forward Euler  FilterMethod=Forward Euler  ControllerParametersSource=internal  P=1  I=0  D=0.5  UseFilter=off  N=100  TunerSelectOption=Transfer Function Based (PID Tuner App)  InitialConditionSource=internal  InitialConditionForIntegrator=0  InitialConditionForFilter=0  DifferentiatorICPrevScaledInput=0  ExternalReset=none  TrackingMode=off  Kt=1  LimitOutput=on  UpperSaturationLimit=deg2rad(20)  LowerSaturationLimit=-deg2rad(20)  LinearizeAsGain=on  AntiWindupMode=clamping  Kb=1  POutMin=[]  POutMax=[]  IOutMin=[]  IOutMax=[]  DOutMin=[]  DOutMax=[]  NOutMin=[]  NOutMax=[]  SumOutMin=[]  SumOutMax=[]  SaturationOutMin=[]  SaturationOutMax=[]  PParamMin=[]  PParamMax=[]  IParamMin=[]  IParamMax=[]  DParamMin=[]  DParamMax=[]  NParamMin=[]  NParamMax=[]  KbParamMin=[]  KbParamMax=[]  KtParamMin=[]  KtParamMax=[]  KbOutMin=[]  KbOutMax=[]  KtOutMin=[]  KtOutMax=[]  IntegratorOutMin=[]  IntegratorOutMax=[]  FilterOutMin=[]  FilterOutMax=[]  SumI1OutMin=[]  SumI1OutMax=[]  SumI2OutMin=[]  SumI2OutMax=[]  SumI3OutMin=[]  SumI3OutMax=[]  SumI4OutMin=[]  SumI4OutMax=[]  SumDOutMin=[]  SumDOutMax=[]  DifferentiatorOutMin=[]  DifferentiatorOutMax=[]  FilterDiffOutCoefMin=[]  FilterDiffOutCoefMax=[]  ReciprocalOutMin=[]  ReciprocalOutMax=[]  SumDenOutMin=[]  SumDenOutMax=[]  SumNumOutMin=[]  SumNumOutMax=[]  DivideOutMin=[]  DivideOutMax=[]  IntegratorContinuousStateAttributes=''  IntegratorStateMustResolveToSignalObject=off  IntegratorRTWStateStorageClass=Auto  FilterContinuousStateAttributes=''  FilterStateMustResolveToSignalObject=off  FilterRTWStateStorageClass=Auto  ParallelPVariant=InternalParameters  IdealPVariant=Disabled  IVariant=InternalParameters  DVariant=InternalParameters  IntegratorVariant=Discrete  SatVariant=Enabled  AWVariant=DiscClampingParallel  PCopyVariant=Disabled  TRVariant=Disabled  FdbkBlocksVariant=Forward  IdealPFdbkVariant=Disabled  SatFdbkVariant=Disabled  DerivativeFilterVariant=Differentiator  NVariant=Passthrough  NCopyVariant=Disabled_SignalSpec  FilterICVariant=InternalICsDifferentiator  IntegratorICVariant=InternalICs  ExternalResetVariant=Disabled  TRSumVariant=Passthrough  SumFdbkVariant=Disabled  SumVariant=Sum_PID
  Saturation5 : Saturate  Commented=on  UpperLimit=0.01*5  LowerLimit=-0.01*5
  Scope : Scope
  Scope20 : Scope  NumInputPorts=3
  Scope22 : Scope  NumInputPorts=3
  Scope23 : Scope  NumInputPorts=2
  Scope6 : Scope  Commented=on  NumInputPorts=2
  Selector : Selector  Commented=on  InputPortWidth=3  IndexOptions=Index vector (dialog)  Indices=[3]  OutputSizes=1
  Signal Specification10 : SignalSpecification  Dimensions=3
  Signal Specification5 : SignalSpecification  Dimensions=4
  Signal Specification6 : SignalSpecification  Dimensions=1
  Signal Specification7 : SignalSpecification  Dimensions=1
  Signal Specification8 : SignalSpecification  Dimensions=1
  Signal Specification9 : SignalSpecification  Dimensions=3
  ZYX-quat : MATLAB Function  TreatAsAtomicUnit=on
  Zero-Order Hold3 : ZeroOrderHold  SampleTime=p.Ts
  q_ref_fly : Outport  VectorParamsAs1DForOutWhenUnconnected=off
  wires:
  MATLAB Function6/1(yawr_slow) -> Signal Specification7/1, Scope22/2, Delay/1, MATLAB Function5/1(yawr)
  Delay1/1 -> MATLAB Function3/1(pitchPID)
  Gain21/1 -> PID Controller1/1
  Signal Specification7/1 -> ZYX-quat/2(z), Scope20/1
  Signal Specification6/1 -> Scope20/2, ZYX-quat/1(y)
  MATLAB Function3/1(vherror) -> Gain21/1
  Signal Specification5/1 -> q_ref_fly/1
  Constant11/1 -> MATLAB Function6/2(maxrate)
  MATLAB Function3/2(pitch) -> Signal Specification6/1
  Zero-Order Hold3/1 -> MATLAB Function8/2(v_wf), MATLAB Function3/3(v_wf)
  MATLAB Function5/1(yawe) -> Scope23/2, PID Controller2/1
  ZYX-quat/1(q) -> Signal Specification5/1
  Signal Specification8/1 -> ZYX-quat/3(x), Scope20/3
  MATLAB Function8/1(yawr) -> MATLAB Function6/1(yawr), Scope22/1
  Signal Specification9/1 -> MATLAB Function8/1(vr_wf), MATLAB Function3/2(vr_wf)
  MATLAB Function8/2(yaw) -> Scope/1, MATLAB Function5/2(yaw)
  v_wf/1 -> Signal Specification10/1
  Delay/1 -> MATLAB Function6/3(yawr_last), Scope22/3
  Signal Specification10/1 -> Zero-Order Hold3/1
  PID Controller2/1 -> Signal Specification8/1, Scope23/1
  PID Controller1/1 -> Delay1/1
  Altitude controller/1 -> Gain/1, Saturation5/1, Scope6/2
  Saturation5/1 -> Scope6/1
  vec2line/1 -> Selector/1
  Selector/1 -> Altitude controller/1
  vr_wf/1 -> Signal Specification9/1
  current_heading/1 -> Delay/2
